simulink model "simu"  (R2017b)
settings: Solver=VariableStepAuto  StartTime=0.0  StopTime=10.0  RelTol=1e-3
settings Model: Creator=ngomi  LastModifiedBy=ngomi

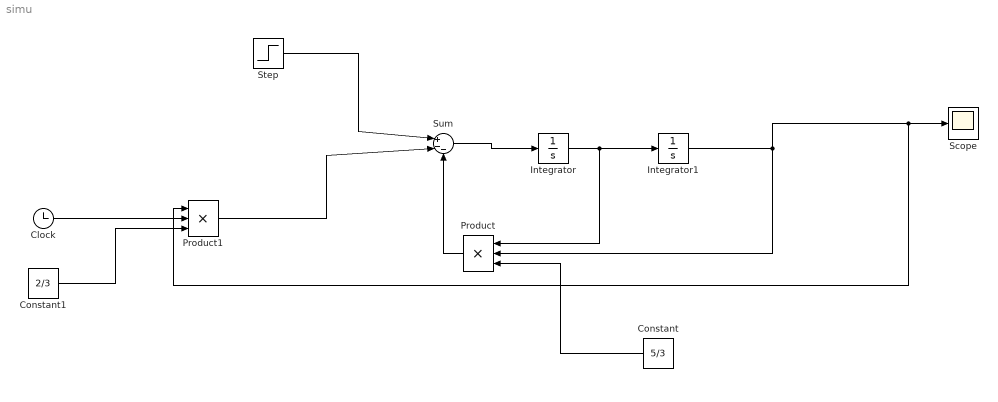
== system simu ==
  Clock : Clock
  Constant : Constant  Value=5/3
  Constant1 : Constant  Value=2/3
  Integrator : Integrator
  Integrator1 : Integrator
  Product : Product  Inputs=3
  Product1 : Product  Inputs=3
  Scope : Scope
  Step : Step  SampleTime=0
  Sum : Sum  Inputs=|+--
  wires:
  Sum/1 -> Integrator/1
  Integrator/1 -> Product/1, Integrator1/1
  Constant/1 -> Product/3
  Product/1 -> Sum/3
  Clock/1 -> Product1/2
  Integrator1/1 -> Scope/1, Product1/1, Product/2
  Constant1/1 -> Product1/3
  Product1/1 -> Sum/2
  Step/1 -> Sum/1
